simulink model "outputregulation"  (R2022a)
settings: Solver=VariableStepAuto  StartTime=0.0  StopTime=10.0  RelTol=1e-3
undefined symbols (not defined in the file or in its folder): A_hat, Aobs, B_hat, Bobs, F_100
settings Model: Creator=user  LastModifiedBy=user

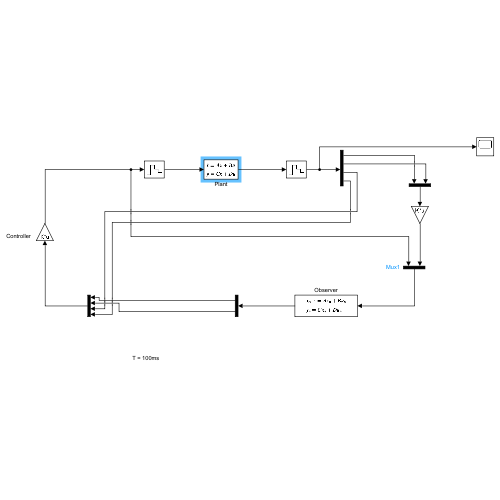
[thumbnail: Simulink's stored preview of the top-level diagram]
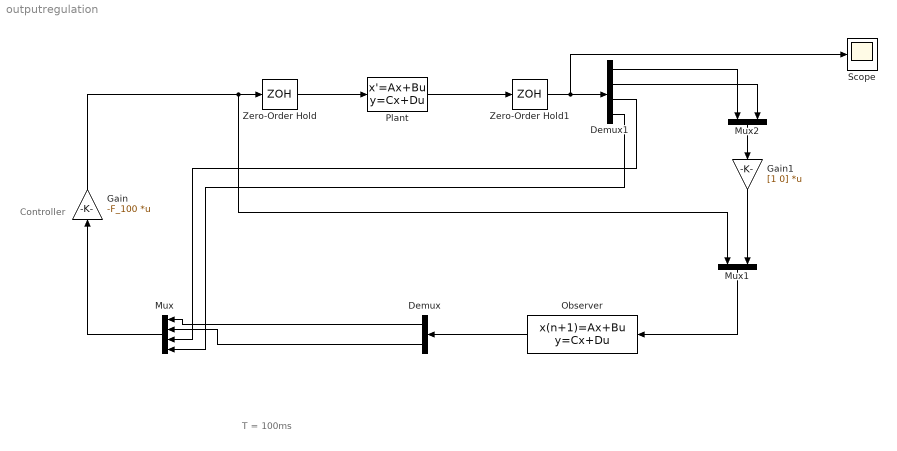
== system outputregulation ==
  note: Controller
  note: T = 100ms
  Demux : Demux  Outputs=2
  Demux1 : Demux
  Gain : Gain  Gain=-F_100  Multiplication=Matrix(K*u)
  Gain1 : Gain  Gain=[1 0]  Multiplication=Matrix(K*u)
  Mux : Mux
  Mux1 : Mux  Inputs=2
  Mux2 : Mux  Inputs=2
  Observer : DiscreteStateSpace  A=Aobs  B=Bobs  C=eye(2)  D=[0 0;0 0]  SampleTime=0.1
  Plant : StateSpace  A=A_hat  B=B_hat  C=eye(4)  D=[0;0;0;0]  InitialCondition=0
  Scope : Scope
  Zero-Order Hold : ZeroOrderHold  SampleTime=0.1
  Zero-Order Hold1 : ZeroOrderHold  SampleTime=0.1
  wires:
  Plant/1 -> Zero-Order Hold1/1
  Mux1/1 -> Observer/1
  Gain/1 -> Mux1/1, Zero-Order Hold/1
  Zero-Order Hold/1 -> Plant/1
  Observer/1 -> Demux/1
  Demux/2 -> Mux/2
  Mux/1 -> Gain/1
  Zero-Order Hold1/1 -> Scope/1, Demux1/1
  Demux1/1 -> Mux2/1
  Demux1/2 -> Mux2/2
  Mux2/1 -> Gain1/1
  Gain1/1 -> Mux1/2
  Demux1/3 -> Mux/3
  Demux1/4 -> Mux/4
  Demux/1 -> Mux/1
